simulink model "APFC_System"  (R2024b)
settings: Solver=VariableStepAuto  StartTime=0.0  StopTime=5  RelTol=1e-3
libraries: spsThreePhaseSeriesRLCLoadLib x4, spsThreePhaseBreakerLib x3, spsThreePhaseSourceLib x1, spsThreePhaseVIMeasurementLib x1, sps_lib x1
settings Model: Creator=vaibh  LastModifiedBy=vaibh

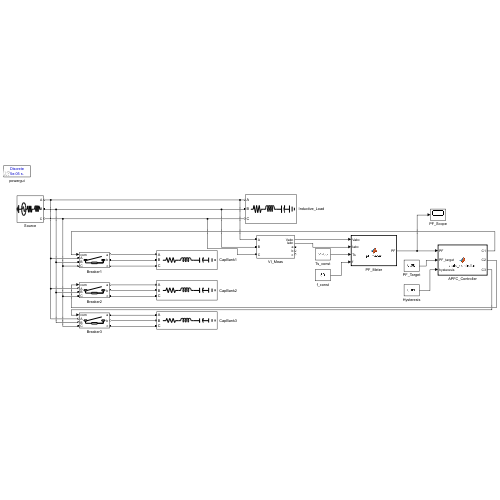
[thumbnail: Simulink's stored preview of the top-level diagram]
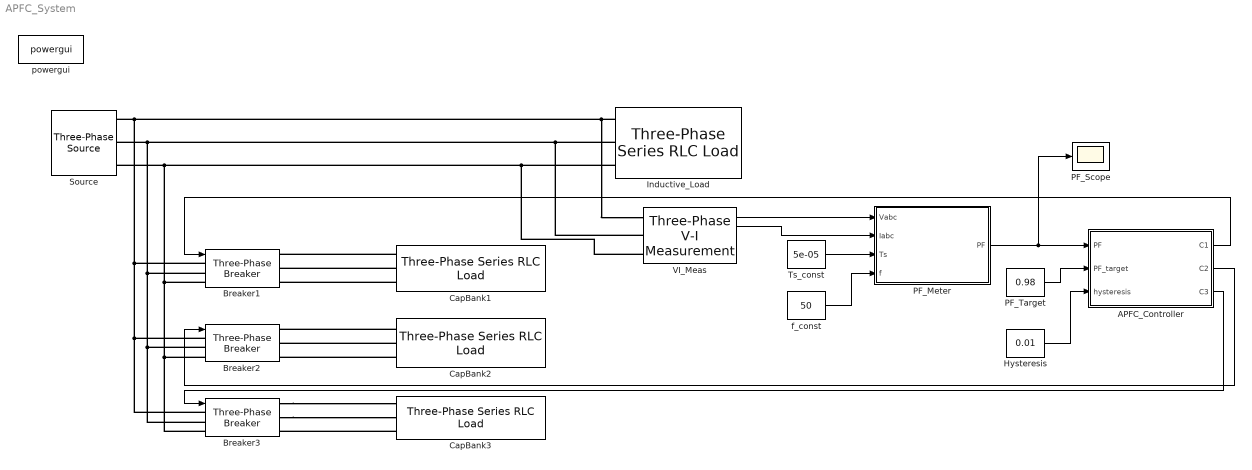
== system APFC_System ==
  APFC_Controller : MATLAB Function  TreatAsAtomicUnit=on
  Breaker1 : spsThreePhaseBreakerLib/Three-Phase Breaker  InitialState=open  SwitchA=on  SwitchB=on  SwitchC=on  SwitchTimes="[1/60  5/60]"  External=on  BreakerResistance=0.01  SnubberResistance=1e6  SnubberCapacitance=inf  Measurements=None
  Breaker2 : spsThreePhaseBreakerLib/Three-Phase Breaker  InitialState=open  SwitchA=on  SwitchB=on  SwitchC=on  SwitchTimes="[1/60  5/60]"  External=on  BreakerResistance=0.01  SnubberResistance=1e6  SnubberCapacitance=inf  Measurements=None
  Breaker3 : spsThreePhaseBreakerLib/Three-Phase Breaker  InitialState=open  SwitchA=on  SwitchB=on  SwitchC=on  SwitchTimes="[1/60  5/60]"  External=on  BreakerResistance=0.01  SnubberResistance=1e6  SnubberCapacitance=inf  Measurements=None
  CapBank1 : spsThreePhaseSeriesRLCLoadLib/Three-Phase Series RLC Load  LConnTagsString=A|B|C  Configuration=Y (grounded)  NominalVoltage=1000  Vabc=[1e3 1e3 1e3]  Vabcp=[1e3 1e3 1e3]  NominalFrequency=60  UnbalancedPower=off  ActivePower=10e3  InductivePower=100  CapacitivePower=100  Pabc=[10e3 9e3 11e3]  QLabc=[100 90 110]  QCabc=[100 90 110]  Pabcp=[10e3 9e3 11e3]  QLabcp=[100 90 110]  QCabcp=[100 90 110]  Measurements=None  LoadType=constant Z
  CapBank2 : spsThreePhaseSeriesRLCLoadLib/Three-Phase Series RLC Load  LConnTagsString=A|B|C  Configuration=Y (grounded)  NominalVoltage=1000  Vabc=[1e3 1e3 1e3]  Vabcp=[1e3 1e3 1e3]  NominalFrequency=60  UnbalancedPower=off  ActivePower=10e3  InductivePower=100  CapacitivePower=100  Pabc=[10e3 9e3 11e3]  QLabc=[100 90 110]  QCabc=[100 90 110]  Pabcp=[10e3 9e3 11e3]  QLabcp=[100 90 110]  QCabcp=[100 90 110]  Measurements=None  LoadType=constant Z
  CapBank3 : spsThreePhaseSeriesRLCLoadLib/Three-Phase Series RLC Load  LConnTagsString=A|B|C  Configuration=Y (grounded)  NominalVoltage=1000  Vabc=[1e3 1e3 1e3]  Vabcp=[1e3 1e3 1e3]  NominalFrequency=60  UnbalancedPower=off  ActivePower=10e3  InductivePower=100  CapacitivePower=100  Pabc=[10e3 9e3 11e3]  QLabc=[100 90 110]  QCabc=[100 90 110]  Pabcp=[10e3 9e3 11e3]  QLabcp=[100 90 110]  QCabcp=[100 90 110]  Measurements=None  LoadType=constant Z
  Hysteresis : Constant  Value=0.01
  Inductive_Load : spsThreePhaseSeriesRLCLoadLib/Three-Phase Series RLC Load  LConnTagsString=A|B|C  Configuration=Y (grounded)  NominalVoltage=1000  Vabc=[1e3 1e3 1e3]  Vabcp=[1e3 1e3 1e3]  NominalFrequency=60  UnbalancedPower=off  ActivePower=10e3  InductivePower=100  CapacitivePower=100  Pabc=[10e3 9e3 11e3]  QLabc=[100 90 110]  QCabc=[100 90 110]  Pabcp=[10e3 9e3 11e3]  QLabcp=[100 90 110]  QCabcp=[100 90 110]  Measurements=None  LoadType=constant Z
  PF_Meter : MATLAB Function  TreatAsAtomicUnit=on
  PF_Scope : Scope
  PF_Target : Constant  Value=0.98
  Source : spsThreePhaseSourceLib/Three-Phase Source  InternalConnection=Yg  VoltagePhases=off  Voltage=415  PhaseAngle=0  Voltage_phases=[25e3 25e3 25e3]/sqrt(3)  PhaseAngles_phases=[0 -120 +120]  Frequency=60  NonIdealSource=on  SpecifyImpedance=off  Resistance=0.8929  Inductance=16.58e-3  ShortCircuitLevel=100e6  BaseVoltage=25e3  XRratio=7  BusType=swing  Pref=10e3  Qref=0  Prefabc=[10e3, 10e3, 10e3]  Qrefabc=[0, 0, 0]  Qmin=-inf  Qmax=inf
  Ts_const : Constant  Value=5e-05
  VI_Meas : spsThreePhaseVIMeasurementLib/Three-Phase V-I Measurement  VoltageMeasurement=phase-to-ground  SetLabelV=off  LabelV=Vabc  Vpu=off  VpuLL=off  CurrentMeasurement=yes  SetLabelI=off  LabelI=Iabc  Ipu=off  Pbase=100e6  Vbase=500e3  OutputType=Complex  PhasorSimulation=off  PSBequivalent=0
  f_const : Constant  Value=50
  powergui : sps_lib/powergui  Priority=1  SimulationMode=Discrete  SampleTime=5e-05  frequency=60  Iterations=50  frequencyindice=60  Pbase=100e6  ErrMax=1e-4  UnitsV=kV  UnitsW=MW  buscounter=0  FunctionMessages=off  echomessages=off  EnableUseOfTLC=off  CurrentSourceSwitches=off  DisableSnubberDevices=off  DisableRonSwitches=off  DisableVfSwitches=off  DisplayEquations=off  AutomaticDiscreteSolvers=off  SolverType=Tustin/Backward Euler (TBE)  Interpol=off  ExternalGateDelay=off  methode=off  Ts=100  x0status=blocks  SPID=on  SwTol=0  HookPort=off  NonlinearTolerance=1e-4  nMaxIteration=100  ContinueOnMaxIteration=off  RestoreLinks=warning  ResistiveCurrentMeasurement=off  Frange=[0:2:500]  Ylog=off  Xlog=on  ShowGrid=off  save=off  variable=ZData  structure=0  ZoomFFT=off  StartTime=0.0  cycles=1  DisplayStyle=1  fundamental=60  FreqAxis=off  MaxFrequency=1000  frequencyindicesteady=1  RmsSteady=1  display=off
  wires:
  VI_Meas/1 -> PF_Meter/1(Vabc)
  VI_Meas/2 -> PF_Meter/2(Iabc)
  Ts_const/1 -> PF_Meter/3(Ts)
  f_const/1 -> PF_Meter/4(f)
  PF_Meter/1(PF) -> PF_Scope/1, APFC_Controller/1(PF)
  PF_Target/1 -> APFC_Controller/2(PF_target)
  Hysteresis/1 -> APFC_Controller/3(hysteresis)
  APFC_Controller/1(C1) -> Breaker1/1
  APFC_Controller/2(C2) -> Breaker2/1
  APFC_Controller/3(C3) -> Breaker3/1
  connections:
  Inductive_Load/LConn1 -- VI_Meas/LConn1 -- Breaker3/LConn1 -- Breaker2/LConn1 -- Breaker1/LConn1 -- Source/RConn1
  Inductive_Load/LConn2 -- VI_Meas/LConn2 -- Breaker3/LConn2 -- Breaker2/LConn2 -- Breaker1/LConn2 -- Source/RConn2
  Inductive_Load/LConn3 -- VI_Meas/LConn3 -- Breaker3/LConn3 -- Breaker2/LConn3 -- Breaker1/LConn3 -- Source/RConn3
  CapBank1/LConn1 -- Breaker1/RConn1
  CapBank1/LConn2 -- Breaker1/RConn2
  CapBank1/LConn3 -- Breaker1/RConn3
  CapBank2/LConn1 -- Breaker2/RConn1
  CapBank2/LConn2 -- Breaker2/RConn2
  CapBank2/LConn3 -- Breaker2/RConn3
  Breaker3/RConn1 -- CapBank3/LConn1
  Breaker3/RConn2 -- CapBank3/LConn2
  CapBank3/LConn3 -- Breaker3/RConn3

== matlab function APFC_System/APFC_Controller ==
  data: PF input; C1 output; PF_target input; hysteresis input; C2 output; C3 output
function [C1,C2,C3] = apfc_controller(PF, PF_target, hysteresis)
persistent stage
if isempty(stage)
    stage = 0;
end
if PF < (PF_target - hysteresis) && stage < 3
    stage = stage + 1;
elseif PF > (PF_target + hysteresis) && stage > 0
    stage = stage - 1;
end
C1 = double(stage >= 1);
C2 = double(stage >= 2);
C3 = double(stage >= 3);
end

== matlab function APFC_System/PF_Meter ==
  data: Vabc input; PF output; Iabc input; Ts input; f input
function PF = pf_meter(Vabc, Iabc, Ts, f)
% Vabc, Iabc: 3-element vectors from the V-I Measurement block's
% Vabc / Iabc signal outputs (set "Output signals" to "Voltages and currents")
persistent bufP bufV2 bufI2 idx bufLen ready
if isempty(idx)
    bufLen = max(round(1/(f*Ts)),1);
    bufP  = zeros(1,bufLen);
    bufV2 = zeros(3,bufLen);
    bufI2 = zeros(3,bufLen);
    idx = 1; ready = false;
end
Vabc = Vabc(:); Iabc = Iabc(:);
bufP(idx)    = sum(Vabc .* Iabc);
bufV2(:,idx) = Vabc.^2;
bufI2(:,idx) = Iabc.^2;
idx = idx + 1;
if idx > bufLen
    idx = 1;
    ready = true;
end
P = mean(bufP);
Vrms = sqrt(mean(bufV2, 2));
Irms = sqrt(mean(bufI2, 2));
S = sum(Vrms .* Irms);
if ready && S > 1e-3
    PF = P / S;
else
    PF = 1;
end
end
